simulink model "sf_elevator"  (Simulink 7.6)
settings: Solver=FixedStepDiscrete  StartTime=0.0  StopTime=inf  FixedStep=0.01  RelTol=1e-3
InitFcn:
  | allCarIds = [1 2];
StartFcn:
  | sf_elevator_gui('init', 'sf_elevator', allCarIds);
StopFcn:
  | sf_elevator_gui('close');
undefined symbols (not defined in the file or in its folder): Stateflow
libraries: sf_elevator_lib x2, sf_gui_elevator_controller_lib x2
CloseFcn:
  | sf_elevator_gui('close');
  | clear allCarIds;
settings Model: Creator=The MathWorks Inc.  CovMetricSettings=dcmtr  ExtModeAutoUpdateStatusClock=off
settings DataIOCC: SaveFormat=StructureWithTime  SignalLoggingName=sigsOut
settings OptimizationCC: InlineInvariantSignals=on  InitFltsAndDblsToZero=on  EfficientMapNaN2IntZero=off  OptimizeModelRefInitCode=on  LifeSpan=Inf
settings DebuggingCC: SaveWithParameterizedLinksMsg=none  SignalResolutionControl=TryResolveAllWithWarning  SolverPrmCheckMsg=none  MultiTaskDSMMsg=warning  MultiTaskCondExecSysMsg=none  StrictBusMsg=None
settings HardwareCC: TargetEndianess=LittleEndian  TargetHWDeviceType=MATLAB Host  ProdEqTarget=off
settings SFSimCC: SFSimEnableDebug=off  SFSimOverflowDetection=off  SFSimEcho=off  SimIntegrity=off  SimParseCustomCode=off
settings RTWCC: SystemTargetFile=ert.tlc  TemplateMakefile=ert_default_tmf  Description=Real-Time Workshop Embedded Coder  GenerateReport=on  ProcessScript=ert_make_rtw_hook  IncludeHyperlinkInReport=on  LaunchReport=on  IncludeERTFirstTime=on  GenerateTraceInfo=on  GenerateTraceReport=on  GenerateTraceReportSl=on  GenerateTraceReportSf=on  GenerateTraceReportEml=on
settings CodeAppCC: IgnoreCustomStorageClasses=off
settings ERTTargetCC: MultiwordLength=2048  GenerateSampleERTMain=on  ERTCustomFileTemplate=example_file_process.tlc  ConvertIfToSwitch=off

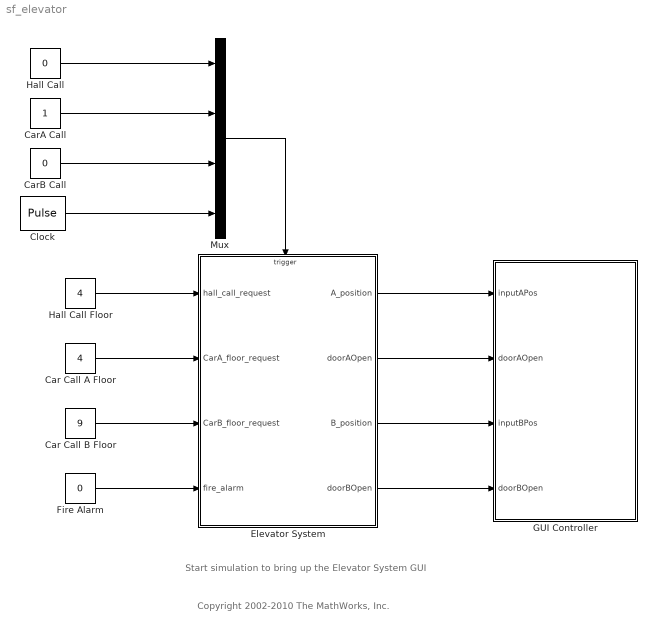
== system sf_elevator ==
  note: Start simulation to bring up the Elevator System GUI
  note: Copyright 2002-2010 The MathWorks, Inc.
  Car Call A Floor : Constant  Value=4  OutDataTypeStr=uint8
  Car Call B Floor : Constant  Value=9  OutDataTypeStr=uint8
  CarA Call : Constant  OutDataTypeStr=double
  CarB Call : Constant  Value=0  OutDataTypeStr=double
  Clock : DiscretePulseGenerator  PulseType=Time based  PulseWidth=50
  Elevator System : Stateflow chart  TreatAsAtomicUnit=on
  Fire Alarm : Constant  Value=0  OutDataTypeStr=boolean
  GUI Controller : Stateflow chart  TreatAsAtomicUnit=on
  Hall Call : Constant  Value=0  OutDataTypeStr=double
  Hall Call Floor : Constant  Value=4  OutDataTypeStr=uint8
  Mux : Mux
  wires:
  Elevator System/1(A_position) -> GUI Controller/1(inputAPos)
  Elevator System/2(doorAOpen) -> GUI Controller/2(doorAOpen)
  Elevator System/3(B_position) -> GUI Controller/3(inputBPos)
  Elevator System/4(doorBOpen) -> GUI Controller/4(doorBOpen)
  Hall Call/1 -> Mux/1
  CarA Call/1 -> Mux/2
  CarB Call/1 -> Mux/3
  Clock/1 -> Mux/4
  Mux/1 -> Elevator System/Trigger
  Hall Call Floor/1 -> Elevator System/1(hall_call_request)
  Car Call A Floor/1 -> Elevator System/2(CarA_floor_request)
  Car Call B Floor/1 -> Elevator System/3(CarB_floor_request)
  Fire Alarm/1 -> Elevator System/4(fire_alarm)

== stateflow chart Elevator System ==
  state Elevator_Manager [parallel]
    settings: executionOrder=1
    state register(hall_call_floor) [function]
      (default) -> (junction 26) : {enqueue(hall_call_floor);
          | hall_call_status[hall_call_floor] = 1;}
    state process_hall_call [function]
      (default) -> (junction 39)
      (junction 39) -> (junction 40) : {
          | /* 'INIT':Initialization */
          | request_floor = hall_call_queue[0];
          | }
      (junction 40) -> (junction 41) : {
          | /* Fire alarm is on */
          | fire_alarm_on = (fire_alarm);
          | }
      (junction 41) -> (junction 42) : {
          | /* There is outstanding request */
          | request_outstanding = (request_floor > 0);
          | }
      (junction 42) -> (junction 43) : {
          | /* Elevator A is idle */
          | elevator_A_idle = (Elevator_A.get_status() == ElevatorStatus.IDLE);
          | }
      (junction 43) -> (junction 44) : {
          | /* Elevator B is idle */
          | elevator_B_idle = (Elevator_B.get_status() == ElevatorStatus.IDLE);
          | }
      (junction 44) -> (junction 45) : {
          | /* Elevator A is closer to request */
          | elevator_A_closer = (fabs(Elevator_A.get_position() - request_floor) <= fabs(Elevator_B.get_position() - request_floor));
          | }
      (junction 45) -> (junction 46) [order 1] : [fire_alarm_on]
      (junction 46) -> (junction 47) : {
          | /* 'EMR':Emergency */
          | Elevator_A.register(floor(Elevator_A.get_position()+Elevator_A.get_direction()/2));
          | Elevator_B.register(floor(Elevator_B.get_position()+Elevator_B.get_direction()/2));
          | }
      (junction 45) -> (junction 48) [order 2]
      (junction 48) -> (junction 49) [order 1] : [!request_outstanding]
      (junction 49) -> (junction 50) : {
          | /* 'NONE':Both elevators are busy, OR no request present */
          |
          | }
      (junction 48) -> (junction 51) [order 2]
      (junction 51) -> (junction 52) [order 1] : [!elevator_A_idle && !elevator_B_idle]
      (junction 52) -> (junction 53) : {
          | /* 'NONE':Both elevators are busy, OR no request present */
          |
          | }
      (junction 51) -> (junction 54) [order 2]
      (junction 54) -> (junction 55) [order 1] : [elevator_A_idle && !elevator_B_idle]
      (junction 55) -> (junction 56) : {
          | /* 'A':Elevator A should respond to request */
          | Elevator_A.enqueue(request_floor);
          | Main_dequeue(request_floor);
          | }
      (junction 54) -> (junction 57) [order 2]
      (junction 57) -> (junction 58) [order 1] : [!elevator_A_idle && elevator_B_idle]
      (junction 58) -> (junction 59) : {
          | /* 'B':Elevator B should respond to request */
          | Elevator_B.enqueue(request_floor);
          | Main_dequeue(request_floor);
          | }
      (junction 57) -> (junction 60) [order 2]
      (junction 60) -> (junction 61) [order 1] : [elevator_A_idle && elevator_B_idle && elevator_A_closer]
      (junction 61) -> (junction 62) : {
          | /* 'A':Elevator A should respond to request */
          | Elevator_A.enqueue(request_floor);
          | Main_dequeue(request_floor);
          | }
      (junction 60) -> (junction 63) [order 2]
      (junction 63) -> (junction 64) [order 1] : [elevator_A_idle && elevator_B_idle && !elevator_A_closer]
      (junction 64) -> (junction 65) : {
          | /* 'B':Elevator B should respond to request */
          | Elevator_B.enqueue(request_floor);
          | Main_dequeue(request_floor);
          | }
      (junction 63) -> (junction 66) [order 2]
    state enqueue(hall_call_floor) [function]
      (junction 23) -> (junction 21) [order 2] : {hall_call_queue[i] = hall_call_floor;}
      (junction 23) -> (junction 22) [order 1] : [i >= NUM_FLOOR]
      (junction 24) -> (junction 23) [order 3]
      (junction 24) -> (junction 24) [order 2] : [hall_call_queue[i] > 0 && i<NUM_FLOOR]{i++;}
      (junction 24) -> (junction 25) [order 1] : [hall_call_queue[i] == hall_call_floor]
      (junction 29) -> (junction 24) [order 2] : {i = 0;}
      (junction 29) -> (junction 28) [order 1] : [hall_call_status[hall_call_floor] != 0]
      (default) -> (junction 29)
    Elevator_Manager -> (junction 35) [order 4] : CLOCK {process_hall_call();} //Clock drives whole system
    Elevator_Manager -> (junction 38) [order 2] : HALL_CALL {register(hall_call_request);}
    Elevator_Manager -> (junction 36) [order 1] : CAR_CALL_B {Elevator_B.register(CarB_floor_request);}
    Elevator_Manager -> (junction 37) [order 3] : CAR_CALL_A  {Elevator_A.register(CarA_floor_request);}
  state Main_dequeue(hall_call_floor) [function]
    (junction 14) -> (junction 13) [order 2]
    (junction 14) -> (junction 15) [order 1] : [i < NUM_FLOOR]
    (junction 15) -> (junction 14) : {hall_call_queue[i] = hall_call_queue[i+1]; i++;}
    (junction 18) -> (junction 15) [order 2]
    (junction 18) -> (junction 17) [order 1] : [i >= NUM_FLOOR || hall_call_queue[i] == 0]
    (junction 20) -> (junction 18) [order 2]
    (junction 20) -> (junction 20) [order 1] : [hall_call_queue[i] > 0 && ...
        | i<NUM_FLOOR && ...
        | hall_call_queue[i] != hall_call_floor]{i++;}
    (default) -> (junction 20) : {i=0;}
  state Elevator_B [parallel]
    settings: executionOrder=3
  state Main_deregister(hall_call_floor) [function]
    (default) -> (junction 34) : {Main_dequeue(hall_call_floor);
        | hall_call_status[hall_call_floor] = 0;}
  state result = Main_exists_in_queue(floor) [function]
    (junction 31) -> (junction 27) [order 2] : {result = i+1;}
    (junction 31) -> (junction 30) [order 1] : [i >= NUM_FLOOR || hall_call_queue[i] == 0]{result = 0;}
    (junction 33) -> (junction 31) [order 2]
    (junction 33) -> (junction 33) [order 1] : [hall_call_queue[i] > 0 && ...
        | i<NUM_FLOOR && ...
        | hall_call_queue[i] != floor]{i++;}
    (default) -> (junction 33) : {i=0;}
  state Elevator_A [parallel]
    settings: executionOrder=2
  data: hall_call_floor function_input double; i temporary uint8; hall_call_floor function_input uint8; request_floor temporary uint8; fire_alarm_on temporary boolean =0; request_outstanding temporary boolean =0; elevator_A_idle temporary boolean =0; elevator_B_idle temporary boolean =0; elevator_A_closer temporary boolean =0; hall_call_floor function_input uint8; i temporary uint8; hall_call_floor function_input uint8; result function_output uint8; floor function_input uint8; i temporary uint8; hall_call_request input uint8; A_position output double =1; NUM_FLOOR constant uint8 =9; CarA_floor_request input uint8; CarB_floor_request input uint8; fire_alarm input boolean; hall_call_queue local uint8 size=10; hall_call_status local uint8 size=10; doorAOpen output boolean =0; B_position output double =1; doorBOpen output boolean =0
  data fire_alarm_on settings: description=Fire alarm is on
  data request_outstanding settings: description=There is outstanding request
  data elevator_A_idle settings: description=Elevator A is idle
  data elevator_B_idle settings: description=Elevator B is idle
  data elevator_A_closer settings: description=Elevator A is closer to request
  events: HALL_CALL input EITHER_EDGE_EVENT; CAR_CALL_A input EITHER_EDGE_EVENT; CAR_CALL_B input EITHER_EDGE_EVENT; CLOCK input EITHER_EDGE_EVENT

== stateflow chart GUI Controller ==
  state CarA_Controller [parallel]
    settings: executionOrder=1
  state CarB_Controller [parallel]
    settings: executionOrder=2
  data: inputAPos input double; doorAOpen input double; inputBPos input double; doorBOpen input double; allCarIds parameter uint8 size=2
